simulink model "Cruise_Control"  (R2020b)
settings: Solver=VariableStepAuto  StartTime=0.0  StopTime=300  RelTol=1e-3
settings Model: Creator=HP  LastModifiedBy=HP

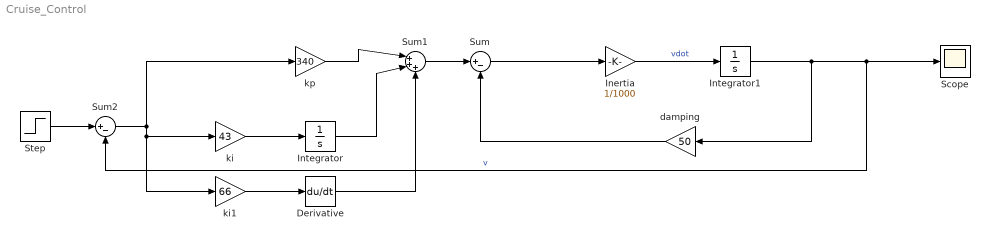
== system Cruise_Control ==
  Derivative : Derivative
  Inertia : Gain  Gain=1/1000
  Integrator : Integrator
  Integrator1 : Integrator
  Scope : Scope
  Step : Step  After=500  SampleTime=0
  Sum : Sum  Inputs=|+-
  Sum1 : Sum  Inputs=|+++
  Sum2 : Sum  Inputs=|+-
  damping : Gain  Gain=50
  ki : Gain  Gain=43
  ki1 : Gain  Gain=66
  kp : Gain  Gain=340
  wires:
  Derivative/1 -> Sum1/3
  Integrator/1 -> Sum1/2
  Sum2/1 -> ki/1, ki1/1, kp/1
  ki1/1 -> Derivative/1
  ki/1 -> Integrator/1
  kp/1 -> Sum1/1
  Integrator1/1 -> Sum2/2, Scope/1, damping/1  "v"
  damping/1 -> Sum/2
  Inertia/1 -> Integrator1/1  "vdot"
  Sum1/1 -> Sum/1
  Sum/1 -> Inertia/1
  Step/1 -> Sum2/1
